simulink model "baseline"  (R2017a)
settings: Solver=VariableStepAuto  StartTime=0.0  StopTime=2  RelTol=1e-3
settings Model: Creator=saturn  LastModifiedBy=saturn

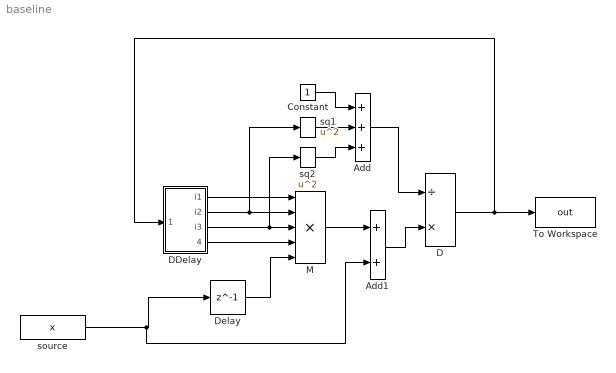
== system baseline ==
  Add : Sum  Inputs=+++
  Add1 : Sum
  Constant : Constant
  D : Product  Inputs=/*
  DDelay : Subsystem
  Delay : Delay  DelayLength=1  InitialCondition=0
  M : Product  Inputs=*****
  To Workspace : ToWorkspace  VariableName=out  SampleTime=-1
      settings: Save2DSignal=2-D array (concatenate along first dimension)
  "source " : FromWorkspace  VariableName=x  SampleTime=0  OutputAfterFinalValue=Setting to zero
  sq1 : Math  Operator=square  SaturateOnIntegerOverflow=on
  sq2 : Math  Operator=square  SaturateOnIntegerOverflow=on
  wires:
  "source "/1 -> Add1/2, Delay/1
  Delay/1 -> M/5
  DDelay/4(i3-1) -> M/4
  DDelay/3(i3) -> sq2/1, M/3
  DDelay/2(i2) -> sq1/1, M/2
  DDelay/1(i1) -> M/1
  sq2/1 -> Add/3
  sq1/1 -> Add/2
  Constant/1 -> Add/1
  Add/1 -> D/1
  D/1 -> DDelay/1(In1), To Workspace/1
  M/1 -> Add1/1
  Add1/1 -> D/2

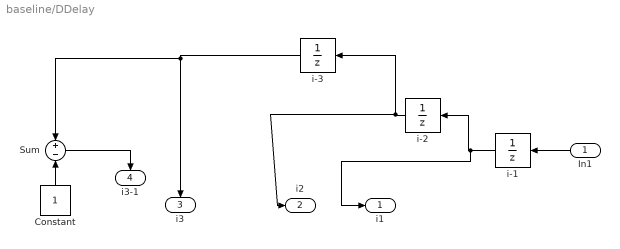
== system baseline/DDelay ==
  In1 : Inport
  Constant : Constant
  Sum : Sum  Inputs=+-
  i-1 : UnitDelay  SampleTime=-1
  i-2 : UnitDelay  SampleTime=-1
  i-3 : UnitDelay  SampleTime=-1
  i1 : Outport
  i2 : Outport  Port=2
  i3 : Outport  Port=3
  i3-1 : Outport  Port=4
  wires:
  i-2/1 -> i-3/1, i2/1
  Constant/1 -> Sum/2
  i-3/1 -> i3/1, Sum/1
  Sum/1 -> i3-1/1
  In1/1 -> i-1/1
  i-1/1 -> i1/1, i-2/1
